simulink model "two_property_tmp"  (Simulink 8.5)
settings: Solver=FixedStepDiscrete  StartTime=0.0  StopTime=10.0  RelTol=1e-3
settings Model: Creator=arnaud  LastModifiedBy=hbourbou  CovSFcnEnable=off
settings DataIOCC: SaveFormat=Structure
settings DebuggingCC: SolverPrmCheckMsg=warning  FcnCallInpInsideContextMsg=EnableAllAsWarning

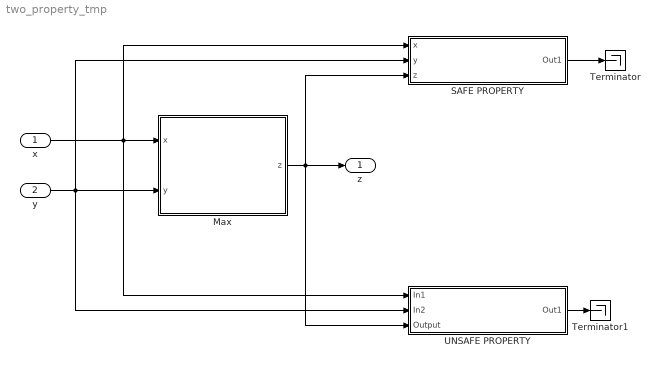
== system two_property_tmp ==
  x : Inport  OutDataTypeStr=int32
  y : Inport  Port=2  OutDataTypeStr=int32
  Max : Subsystem
  SAFE PROPERTY : Subsystem  TreatAsAtomicUnit=on  mask(Observer){AnnotationType=ensures, ObserverType=ellipsoid}
      mask prompts: AnnotationType "Type of annotation (pre/post...)"; ObserverType "Observer type"
      mask help:
      | Set an observer for the system.
      | The annotation type parameter sets the type of observer:
      | - requires : pre-condition
      | - ensures : post-condition
      | - assert : an assertion
      | - observer : the observer computes a special type of properties
      mask TypeOptions AnnotationType: ensures | requires | assert | observer
      mask Callback AnnotationType:
      | paramStr = get_param(gcb, 'MaskValues');
      | 
      | if strcmp(paramStr{1}(1),'o')
      |     set_param(gcb,'MaskVisibilities',{'on';'on'});
      |     paramStr{2} = 'ellipsoid';
      |     set_param(gcb,'MaskValues',paramStr);
      | else
      |     set_param(gcb,'MaskVisibilities',{'on';'off'});
      | end
      mask Callback ObserverType:
      | paramStr = get_param(gcb, 'MaskValues');
      | 
      | if strcmp(paramStr{1}(1),'observer')
      |     set_param(gcb,'MaskVisibilities',{'on';'on'});
      |     paramStr{2} = 'ellipsoid';
      |     set_param(gcb,'MaskValues',paramStr);
      | else
      |     set_param(gcb,'MaskVisibilities',{'on';'off'});
      | end
      mask Display:
      | color('red')
      | text(0.5, 0.5, 'Observer Block', 'horizontalAlignment', 'center');
  Terminator : Terminator
  Terminator1 : Terminator
  UNSAFE PROPERTY : Subsystem  TreatAsAtomicUnit=on  mask(Observer){AnnotationType=ensures, ObserverType=ellipsoid}
      mask prompts: AnnotationType "Type of annotation (pre/post...)"; ObserverType "Observer type"
      mask help:
      | Set an observer for the system.
      | The annotation type parameter sets the type of observer:
      | - requires : pre-condition
      | - ensures : post-condition
      | - assert : an assertion
      | - observer : the observer computes a special type of properties
      mask TypeOptions AnnotationType: ensures | requires | assert | observer
      mask Callback AnnotationType:
      | paramStr = get_param(gcb, 'MaskValues');
      | 
      | if strcmp(paramStr{1}(1),'o')
      |     set_param(gcb,'MaskVisibilities',{'on';'on'});
      |     paramStr{2} = 'ellipsoid';
      |     set_param(gcb,'MaskValues',paramStr);
      | else
      |     set_param(gcb,'MaskVisibilities',{'on';'off'});
      | end
      mask Callback ObserverType:
      | paramStr = get_param(gcb, 'MaskValues');
      | 
      | if strcmp(paramStr{1}(1),'observer')
      |     set_param(gcb,'MaskVisibilities',{'on';'on'});
      |     paramStr{2} = 'ellipsoid';
      |     set_param(gcb,'MaskValues',paramStr);
      | else
      |     set_param(gcb,'MaskVisibilities',{'on';'off'});
      | end
      mask Display:
      | color('red')
      | text(0.5, 0.5, 'Observer Block', 'horizontalAlignment', 'center');
  z : Outport
  wires:
  x/1 -> UNSAFE PROPERTY/1(In1), Max/1(x), SAFE PROPERTY/1(x)
  y/1 -> Max/2(y), UNSAFE PROPERTY/2(In2), SAFE PROPERTY/2(y)
  SAFE PROPERTY/1(Out1) -> Terminator/1
  UNSAFE PROPERTY/1(Out1) -> Terminator1/1
  Max/1(z) -> SAFE PROPERTY/3(z), z/1, UNSAFE PROPERTY/3(Output)

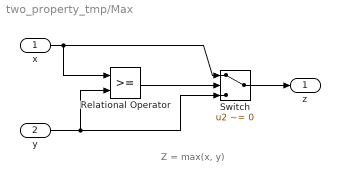
== system two_property_tmp/Max ==
  note: Z = max(x, y)
  x : Inport
  y : Inport  Port=2
  Relational Operator : RelationalOperator  OutDataTypeStr=boolean
  Switch : Switch  Criteria=u2 ~= 0
  z : Outport
  wires:
  Relational Operator/1 -> Switch/2
  Switch/1 -> z/1
  x/1 -> Relational Operator/1, Switch/1
  y/1 -> Switch/3, Relational Operator/2

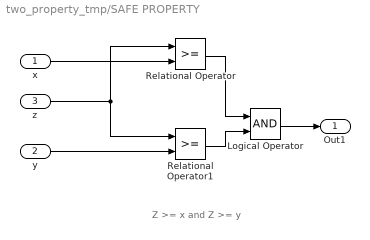
== system two_property_tmp/SAFE PROPERTY ==
  note: Z >= x and Z >= y
  x : Inport
  y : Inport  Port=2
  z : Inport  Port=3
  Logical Operator : Logic  AllPortsSameDT=off  OutDataTypeStr=boolean
  Relational Operator : RelationalOperator  OutDataTypeStr=boolean
  Relational Operator1 : RelationalOperator  OutDataTypeStr=boolean
  Out1 : Outport
  wires:
  Relational Operator/1 -> Logical Operator/1
  Relational Operator1/1 -> Logical Operator/2
  Logical Operator/1 -> Out1/1
  z/1 -> Relational Operator/1, Relational Operator1/1
  x/1 -> Relational Operator/2
  y/1 -> Relational Operator1/2

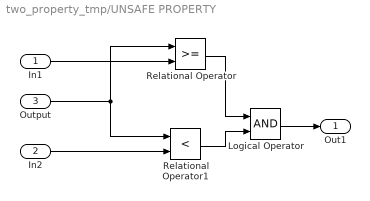
== system two_property_tmp/UNSAFE PROPERTY ==
  In1 : Inport
  In2 : Inport  Port=2
  Output : Inport  Port=3
  Logical Operator : Logic  AllPortsSameDT=off  OutDataTypeStr=boolean
  Relational Operator : RelationalOperator  OutDataTypeStr=boolean
  Relational Operator1 : RelationalOperator  Operator=<  OutDataTypeStr=boolean
  Out1 : Outport
  wires:
  Relational Operator/1 -> Logical Operator/1
  Relational Operator1/1 -> Logical Operator/2
  Logical Operator/1 -> Out1/1
  Output/1 -> Relational Operator/1, Relational Operator1/1
  In1/1 -> Relational Operator/2
  In2/1 -> Relational Operator1/2
